simulink model "INCMPPT"  (R2014b)
settings: Solver=ode45  StartTime=0.0  StopTime=2  RelTol=1e-3
undefined symbols (not defined in the file or in its folder): sigbuilder_block
libraries: powerlib x14, powerlib_meascontrol x1
settings Model: Creator=nitukeee  LastModifiedBy=nitukeee

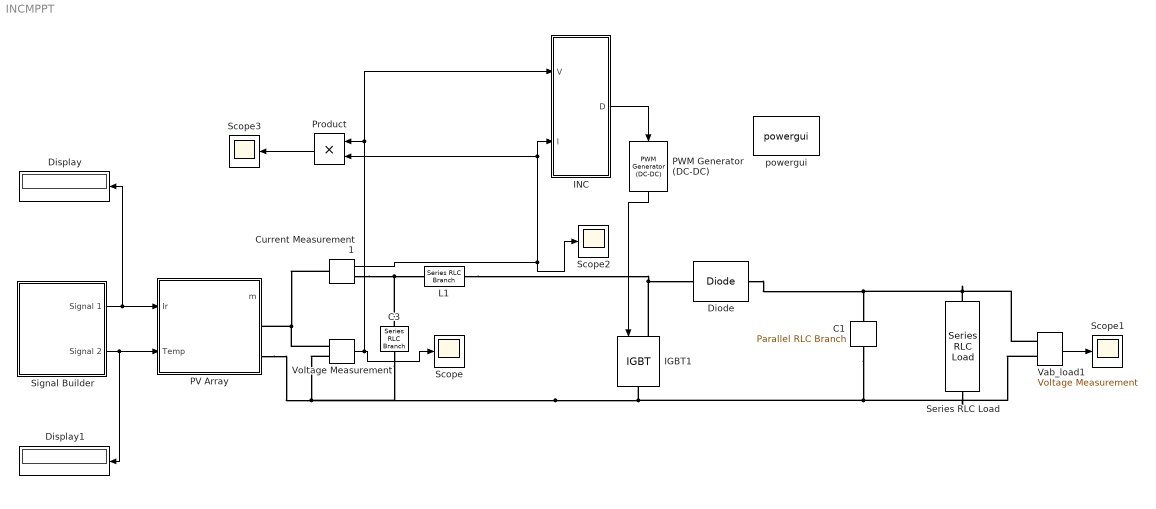
== system INCMPPT ==
  C1 : powerlib/Elements/Parallel RLC Branch  LConnTagsString=a  RConnTagsString=__new0  BranchType=C  Resistance=1  Inductance=1e-3  SetiL0=off  InitialCurrent=0  Capacitance=12000e-6  Setx0=off  InitialVoltage=0  Measurements=None
  C3 : powerlib/Elements/Series RLC Branch  LConnTagsString=__new0  RConnTagsString=__new0  BranchType=C  Resistance=1  Inductance=1e-3  SetiL0=off  InitialCurrent=0  Capacitance=100e-6  Setx0=off  InitialVoltage=0  Measurements=None
  Current Measurement1 : powerlib/Measurements/Current Measurement  PhasorSimulation=off  OutputType=Complex  PSBequivalent=0
  Diode : powerlib/Power Electronics/Diode  Ron=0.001  Lon=0  Vf=0.8  IC=0  UseSnubber=off  Rs=500  Cs=250e-9  Measurements=off
  Display : Display
  Display1 : Display
  IGBT1 : powerlib/Power Electronics/IGBT  Ron=0.001  Lon=0  Vf=1  Tf=1e-6  Tt=2e-6  IC=0  Rs=1e5  Cs=inf  Measurements=off
  INC : Subsystem
  L1 : powerlib/Elements/Series RLC Branch  LConnTagsString=__new0  RConnTagsString=__new0  BranchType=RL  Resistance=0.005  Inductance=0.005  SetiL0=off  InitialCurrent=0  Capacitance=1e-6  Setx0=off  InitialVoltage=0  Measurements=None
  PV Array : Subsystem  mask(PV array){ModuleType=SunPower SPR-305-WHT, Ncell=96, Nser=5, Npar=66, Voc=64.2, Isc=5.96, Vm=54.7, Im=5.58, TempC_Voc=-0.177, TempC_Isc=0.003516, TempC_Vmp=-0.186, TempC_Imp=-0.00212, Qd=1.25, Temperature=[0   25   50   75  100], Iph_Temp=[5.9045      5.9606      6.0494      6.1386      6.2292], Isat_Temp=[1.6236e-10  5.2622e-09  9.8888e-08  1.2201e-06  1.0769e-05], Rp_Temp=[1723.2701      819.13001       313.3225      186.86379      130.70398], Rs_Temp=[0.10187    0.083029    0.075997    0.085738      0.1163], PlotVI_module=off, PlotVI_array=off, PlotVI_array_Temp=off, Ts=1e-6}
      mask prompts: ModuleType "Module type:"; Ncell "Number of cells per module:"; Nser "Number of series-connected  modules per string (Nser):"; Npar "Number of parallel strings (Npar):"; Voc "Open circuit voltage  Voc (V):"; Isc "Short-circuit current Isc (A):"; Vm "Voltage at maximum power point Vmp (V):"; Im "Current at maximum power point Imp (A):"; TempC_Voc "Temperature coefficient of Voc (V/deg.C)"; TempC_Isc "Temperature coefficient of Isc (A/deg.C)"; TempC_Vmp "Temperature coefficient of Vmp (V/deg.C)"; TempC_Imp "Temperature coefficient of Imp (A/deg.C"; Qd "Diode Quality factor"; Temperature "Cell temperature (degrees C)"; Iph_Temp "Photo-current source Iph  (A):"; Isat_Temp "Diode saturation current Isat (A):"; Rp_Temp "Parallel resistance Rp (ohms):"; Rs_Temp "Series resistance Rs (ohms):"; PlotVI_module "Display  I-V and  P-V characteristics of one module at 25 deg.C"; PlotVI_array "Display  I-V and  P-V characteristics of array at 25 deg.C"; PlotVI_array_Temp "Display  I-V and  P-V char. of array at 100W/m^2  for specified temperatures"; Ts "Sample time"
      mask help:
      | Model a PV array.
      |
      | PV array consists of Npar strings of modules connected in parallel, each string consisting of Nser modules connected in series.
      |
      | Input 1 = Sun irradiance (W/m^2)
      | Input 2 = Cell temperature (deg.C))
      |
      | Module specifications provided by manufacturer (Voc, Isc, Vmp, Imp) as well as temperature coefficients are listed under 'Module' Tab.
      | The four PV model parameters for one module (photo-generated current Iph, diode saturation current Isat, parallel resistance Rp and  series resistance Rs) are listed under the 'Model' Tab. These parameters are adusted to fit Voc, Isc, Vmp, Imp at specied cell temperatures listed under 'Module' Tab and assuming a given "diode quality factor" (Qd) for the semiconductor.
      |
      | Select a 'Module type' and then press Apply to see module parameters.
      | Note: Module characteristics are extracted from NREL System Advisor Model.
      mask init:
      | BlockName=gcb;
      | 
      | % Solar Modules Specifications
      | %=============================
      | %
      | Type=1;
      | SolarModuleSpec(Type).Desc= 'Kyocera KD135GX-LP';
      | SolarModuleSpec(Type).nCells= 36;
      | SolarModuleSpec(Type).Voc= 22.0999;
      | SolarModuleSpec(Type).Isc= 8.36955;
      | SolarModuleSpec(Type).Vmp= 17.7;
      | SolarModuleSpec(Type).Imp= 7.62959;
      | SolarModuleSpec(Type).TempC_Voc= -0.08;
      | SolarModuleSpec(Type).TempC_Isc= 0.005022;
      | SolarModuleSpec(Type).TempC_Vmp= -0.082;
      | SolarModuleSpec(Type).TempC_Imp= -0.001068;
      | SolarModuleSpec(Type).TempC= [0   25   50   75  100];
      | SolarModuleSpec(Type).Qd= 1.25;
      | SolarModuleSpec(Type).Iph= [8.2548      8.3863      8.5179      8.6475      8.7657];
      | SolarModuleSpec(Type).Isat= [1.0452e-09  4.0088e-08  8.7854e-07   1.246e-05  0.00012585];
      | SolarModuleSpec(Type).Rp= [124.2147      80.21788      61.82143      57.59975       93.2949];
      | SolarModuleSpec(Type).Rs= [0.16273     0.16086     0.16567     0.17914     0.20462];
      | SolarModuleSpec(Type).VT= [1.0586      1.1555      1.2525      1.3494      1.4463];
      | 
      | Type=2;
      | SolarModuleSpec(Type).Desc= 'Kyocera KD205GX-LP';
      | SolarModuleSpec(Type).nCells= 54;
      | SolarModuleSpec(Type).Voc= 33.1999;
      | SolarModuleSpec(Type).Isc= 8.35955;
      | SolarModuleSpec(Type).Vmp= 26.6;
      | SolarModuleSpec(Type).Imp= 7.70959;
      | SolarModuleSpec(Type).TempC_Voc= -0.12;
      | SolarModuleSpec(Type).TempC_Isc= 0.005016;
      | SolarModuleSpec(Type).TempC_Vmp= -0.123;
      | SolarModuleSpec(Type).TempC_Imp= -0.001079;
      | SolarModuleSpec(Type).TempC= [0   25   50   75  100];
      | SolarModuleSpec(Type).Qd= 1.5;
      | SolarModuleSpec(Type).Iph= [8.2611      8.3642      8.4897      8.6397      8.8494];
      | SolarModuleSpec(Type).Isat= [4.6184e-08  9.7399e-07  1.2856e-05  0.00011784  0.00080899];
      | SolarModuleSpec(Type).Rp= [1053.4598       1010.571      746.03259      733.82072      575.51725];
      | SolarModuleSpec(Type).Rs= [0.16179     0.15945     0.16818     0.19126     0.23373];
      | SolarModuleSpec(Type).VT= [1.9055      2.0799      2.2544      2.4289      2.6034];
      | 
      | Type=3;
      | SolarModuleSpec(Type).Desc= 'Mitsubishi PV-UD190MF5';
      | SolarModuleSpec(Type).nCells= 50;
      | SolarModuleSpec(Type).Voc= 30.8006;
      | SolarModuleSpec(Type).Isc= 8.23289;
      | SolarModuleSpec(Type).Vmp= 24.6999;
      | SolarModuleSpec(Type).Imp= 7.71272;
      | SolarModuleSpec(Type).TempC_Voc= -0.105;
      | SolarModuleSpec(Type).TempC_Isc= 0.004446;
      | SolarModuleSpec(Type).TempC_Vmp= -0.109;
      | SolarModuleSpec(Type).TempC_Imp= -0.0007713;
      | SolarModuleSpec(Type).TempC= [0   25   50   75  100];
      | SolarModuleSpec(Type).Qd= 1.25;
      | SolarModuleSpec(Type).Iph= [8.1758      8.2585      8.3644      8.4965      8.6704];
      | SolarModuleSpec(Type).Isat= [1.0882e-09  3.8061e-08  7.7001e-07  1.0166e-05  9.5622e-05];
      | SolarModuleSpec(Type).Rp= [760.17338      1011.1501      920.18116      953.25748       1044.703];
      | SolarModuleSpec(Type).Rs= [0.22154      0.2231     0.23302     0.25351     0.28829];
      | SolarModuleSpec(Type).VT= [1.4703      1.6049      1.7395      1.8742      2.0088];
      | 
      | Type=4;
      | SolarModuleSpec(Type).Desc= 'Sanyo HIP-225HDE1';
      | SolarModuleSpec(Type).nCells= 60;
      | SolarModuleSpec(Type).Voc= 41.7984;
      | SolarModuleSpec(Type).Isc= 7.13383;
      | SolarModuleSpec(Type).Vmp= 33.9;
      | SolarModuleSpec(Type).Imp= 6.63419;
      | SolarModuleSpec(Type).TempC_Voc= -0.105;
      | SolarModuleSpec(Type).TempC_Isc= 0.00214;
      | SolarModuleSpec(Type).TempC_Vmp= -0.101;
      | SolarModuleSpec(Type).TempC_Imp= -0.0006634;
      | SolarModuleSpec(Type).TempC= [0   25   50   75  100];
      | SolarModuleSpec(Type).Qd= 1.75;
      | SolarModuleSpec(Type).Iph= [7.1125      7.1668      7.2277      7.3002      7.3835];
      | SolarModuleSpec(Type).Isat= [1.0956e-07   1.322e-06  1.0873e-05  6.6227e-05  0.00031754];
      | SolarModuleSpec(Type).Rp= [1677.488      1798.4952      1967.0424      1956.9124      2053.1618];
      | SolarModuleSpec(Type).Rs= [0.19173     0.14196     0.10096    0.069476    0.049098];
      | SolarModuleSpec(Type).VT= [2.47      2.6962      2.9224      3.1486      3.3748];
      | 
      | Type=5;
      | SolarModuleSpec(Type).Desc= 'SunPower SPR-305-WHT';
      | SolarModuleSpec(Type).nCells= 96;
      | SolarModuleSpec(Type).Voc= 64.2;
      | SolarModuleSpec(Type).Isc= 5.96;
      | SolarModuleSpec(Type).Vmp= 54.7;
      | SolarModuleSpec(Type).Imp= 5.58;
      | SolarModuleSpec(Type).TempC_Voc= -0.177;
      | SolarModuleSpec(Type).TempC_Isc= 0.003516;
      | SolarModuleSpec(Type).TempC_Vmp= -0.186;
      | SolarModuleSpec(Type).TempC_Imp= -0.00212;
      | SolarModuleSpec(Type).TempC= [0   25   50   75  100];
      | SolarModuleSpec(Type).Qd= 1.25;
      | SolarModuleSpec(Type).Iph= [5.9045      5.9606      6.0494      6.1386      6.2292];
      | SolarModuleSpec(Type).Isat= [1.6236e-10  5.2622e-09  9.8888e-08  1.2201e-06  1.0769e-05];
      | SolarModuleSpec(Type).Rp= [1723.2701      819.13001       313.3225      186.86379      130.70398];
      | SolarModuleSpec(Type).Rs= [0.10187    0.083029    0.075997    0.085738      0.1163];
      | SolarModuleSpec(Type).VT= [2.8229      3.0814      3.3399      3.5984      3.8569];
      | 
      | Type=6;
      | SolarModuleSpec(Type).Desc= 'Suntech STP270S-24_Vb';
      | SolarModuleSpec(Type).nCells= 72;
      | SolarModuleSpec(Type).Voc= 44.4999;
      | SolarModuleSpec(Type).Isc= 8.19978;
      | SolarModuleSpec(Type).Vmp= 35;
      | SolarModuleSpec(Type).Imp= 7.70979;
      | SolarModuleSpec(Type).TempC_Voc= -0.1504;
      | SolarModuleSpec(Type).TempC_Isc= 0.004969;
      | SolarModuleSpec(Type).TempC_Vmp= -0.1567;
      | SolarModuleSpec(Type).TempC_Imp= 0.0001234;
      | SolarModuleSpec(Type).TempC= [0   25   50   75  100];
      | SolarModuleSpec(Type).Qd= 1.25;
      | SolarModuleSpec(Type).Iph= [8.1345      8.2466      8.3792      8.5437      8.7583];
      | SolarModuleSpec(Type).Isat= [1.0212e-09   3.569e-08  7.2273e-07  9.5489e-06  8.9954e-05];
      | SolarModuleSpec(Type).Rp= [1505.3115      1827.4593      2300.9307      2164.0121      1763.1975];
      | SolarModuleSpec(Type).Rs= [0.4218     0.42722     0.44553     0.48023      0.5376];
      | SolarModuleSpec(Type).VT= [2.1172      2.3111      2.5049      2.6988      2.8927];
      | 
      | Type=7;
      | SolarModuleSpec(Type).Desc= 'Canadian Solar CS5P-220M';
      | SolarModuleSpec(Type).nCells= 96;
      | SolarModuleSpec(Type).Voc= 59.2618;
      | SolarModuleSpec(Type).Isc= 5.09261;
      | SolarModuleSpec(Type).Vmp= 48.3159;
      | SolarModuleSpec(Type).Imp= 4.54758;
      | SolarModuleSpec(Type).TempC_Voc= -0.217;
      | SolarModuleSpec(Type).TempC_Isc= 0.002022;
      | SolarModuleSpec(Type).TempC_Vmp= -0.2355;
      | SolarModuleSpec(Type).TempC_Imp= 0.0008231;
      | SolarModuleSpec(Type).TempC= [0   25   50   75  100];
      | SolarModuleSpec(Type).Qd= 1.5;
      | SolarModuleSpec(Type).Iph= [5.046       5.098      5.1493      5.1959      5.3427];
      | SolarModuleSpec(Type).Isat= [2.4207e-08  5.3103e-07  7.2907e-06  6.9747e-05  0.00049283];
      | SolarModuleSpec(Type).Rp= [222.52442      235.76261      303.25525      1307.0023      2378.4408];
      | SolarModuleSpec(Type).Rs= [0.17441     0.24807     0.36157     0.52616      0.7509];
      | SolarModuleSpec(Type).VT= [3.3875      3.6977      4.0079      4.3181      4.6283];
      | 
      | Type=8;
      | SolarModuleSpec(Type).Desc= 'BP Solar SX3190';
      | SolarModuleSpec(Type).nCells= 50;
      | SolarModuleSpec(Type).Voc= 30.6021;
      | SolarModuleSpec(Type).Isc= 8.51029;
      | SolarModuleSpec(Type).Vmp= 24.3003;
      | SolarModuleSpec(Type).Imp= 7.82945;
      | SolarModuleSpec(Type).TempC_Voc= -0.111;
      | SolarModuleSpec(Type).TempC_Isc= 0.005532;
      | SolarModuleSpec(Type).TempC_Vmp= -0.114;
      | SolarModuleSpec(Type).TempC_Imp= -0.001566;
      | SolarModuleSpec(Type).TempC= [0   25   50   75  100];
      | SolarModuleSpec(Type).Qd= 1.25;
      | SolarModuleSpec(Type).Iph= [8.3797      8.5214       8.667      8.8096      8.9362];
      | SolarModuleSpec(Type).Isat= [1.1494e-09  4.3763e-08   9.524e-07  1.3432e-05  0.00013518];
      | SolarModuleSpec(Type).Rp= [479.1668      189.6748      120.6956      107.8176      267.7255];
      | SolarModuleSpec(Type).Rs= [0.24905     0.24841     0.25704     0.27792     0.31611];
      | SolarModuleSpec(Type).VT= [1.4703      1.6049      1.7395      1.8742      2.0088];
      | 
      | Type=9;
      | SolarModuleSpec(Type).Desc= 'First Solar FS-272';
      | SolarModuleSpec(Type).nCells= 116;
      | SolarModuleSpec(Type).Voc= 94.5738;
      | SolarModuleSpec(Type).Isc= 1.18103;
      | SolarModuleSpec(Type).Vmp= 70.558;
      | SolarModuleSpec(Type).Imp= 1.01088;
      | SolarModuleSpec(Type).TempC_Voc= -0.269;
      | SolarModuleSpec(Type).TempC_Isc= 0.0005433;
      | SolarModuleSpec(Type).TempC_Vmp= -0.206;
      | SolarModuleSpec(Type).TempC_Imp= -0.0003538;
      | SolarModuleSpec(Type).TempC= [0   25   50   75  100];
      | SolarModuleSpec(Type).Qd= 3;
      | SolarModuleSpec(Type).Iph= [1.1706      1.1841      1.1969       1.209      1.2204];
      | SolarModuleSpec(Type).Isat= [4.7807e-06   2.871e-05  0.00013082  0.00048055    0.001489];
      | SolarModuleSpec(Type).Rp= [2555.993      1859.5401      1459.3976      1213.5712      1072.4965];
      | SolarModuleSpec(Type).Rs= [6.9861      4.7977      2.7078     0.74048           0];
      | SolarModuleSpec(Type).VT= [8.1864      8.93607      9.68574      10.4354      11.1851];
      | 
      | Type=10;
      | SolarModuleSpec(Type).Desc= 'SunPower 128-cell Module';
      | SolarModuleSpec(Type).nCells= 128;
      | SolarModuleSpec(Type).Voc= 85.2983;
      | SolarModuleSpec(Type).Isc= 5.8675;
      | SolarModuleSpec(Type).Vmp= 72.8992;
      | SolarModuleSpec(Type).Imp= 5.48769;
      | SolarModuleSpec(Type).TempC_Voc= -0.2664;
      | SolarModuleSpec(Type).TempC_Isc= 0.001837;
      | SolarModuleSpec(Type).TempC_Vmp= -0.276;
      | SolarModuleSpec(Type).TempC_Imp= -0.00169;
      | SolarModuleSpec(Type).TempC= [0   25   50   75  100];
      | SolarModuleSpec(Type).Qd= 1.5;
      | SolarModuleSpec(Type).Iph= [5.8403      5.8693      5.9126      5.9583      6.0069];
      | SolarModuleSpec(Type).Isat= [8.3639e-09  1.7905e-07  2.3847e-06  2.1965e-05  0.00015113];
      | SolarModuleSpec(Type).Rp= [3739.8323      3390.2471      1695.8516      1327.4043      1910.4252];
      | SolarModuleSpec(Type).Rs= [0  0  0  0  0];
      | SolarModuleSpec(Type).VT= [4.5166      4.9302      5.3439      5.7575      6.1711];
      | 
      | 
      | %-------------------------------------------------------------------------
      | 
      | Type=strmatch(ModuleType,char(SolarModuleSpec.Desc));
      | 
      | % Write module prameters inside mask
      | %===================================
      | set_param(BlockName,'Ncell',num2str(SolarModuleSpec(Type).nCells));
      | set_param(BlockName,'Voc',num2str(SolarModuleSpec(Type).Voc));
      | set_param(BlockName,'Isc',num2str(SolarModuleSpec(Type).Isc));
      | set_param(BlockName,'Vm',num2str(SolarModuleSpec(Type).Vmp));
      | set_param(BlockName,'Im',num2str(SolarModuleSpec(Type).Imp));
      | set_param(BlockName,'TempC_Voc',num2str(SolarModuleSpec(Type).TempC_Voc));
      | set_param(BlockName,'TempC_Isc',num2str(SolarModuleSpec(Type).TempC_Isc));
      | set_param(BlockName,'TempC_Vmp',num2str(SolarModuleSpec(Type).TempC_Vmp));
      | set_param(BlockName,'TempC_Imp',num2str(SolarModuleSpec(Type).TempC_Imp));
      | 
      | set_param(BlockName,'Qd',num2str(SolarModuleSpec(Type).Qd));
      | 
      | set_param(BlockName,'Temperature',['[',num2str(SolarModuleSpec(Type).TempC),']']);
      | set_param(BlockName,'Iph_Temp',['[',num2str(SolarModuleSpec(Type).Iph),']']);
      | set_param(BlockName,'Isat_Temp',['[',num2str(SolarModuleSpec(Type).Isat),']']);
      | set_param(BlockName,'Rp_Temp',['[',num2str(SolarModuleSpec(Type).Rp),']']);
      | set_param(BlockName,'Rs_Temp',['[',num2str(SolarModuleSpec(Type).Rs),']']);
      | 
      | TC=25; % standard test temperature (deg. C)
      | T=273+TC; %(Kelvin)
      | nT=find(SolarModuleSpec(Type).TempC==TC);
      | 
      | % Array model parameters
      | %=======================
      | % Qd=SolarModuleSpec(Type).Qd;
      | % k= 1.3806e-23; % Boltzman constant (J.K^-1)
      | % q=1.6022e-19;  % electron charge  (C)
      | % VT=k*T/q*nCells*Qd;
      | VT=SolarModuleSpec(Type).VT(nT);Iph=SolarModuleSpec(Type).Iph(nT); 
      | 
      | TempC=SolarModuleSpec(Type).TempC;
      | Iph_array=SolarModuleSpec(Type).Iph*Npar;
      | Isat_array=SolarModuleSpec(Type).Isat*Npar;
      | VT_array=SolarModuleSpec(Type).VT*Nser;
      | Rs_array=SolarModuleSpec(Type).Rs*Nser/Npar;
      | Rp_array=SolarModuleSpec(Type).Rp*Nser/Npar;
      | 
      | % Used to determine initial value of Boost Control (MPPT)
      | % assignin('base','Vm_Init',Vm*Nser);
      | %
      | % Plot module and array I-V & P-V characteristics for different irradiances
      | % =========================================================================
      | if PlotVI_module || PlotVI_array 
      |     Voc=SolarModuleSpec(Type).Voc; 
      |     Isc=SolarModuleSpec(Type).Isc; 
      |     Vm=SolarModuleSpec(Type).Vmp;  
      |     Im=SolarModuleSpec(Type).Imp;
      |     
      |     load_system('PV_model_Param');
      |     
      |     assignin('base','Voc',Voc);
      |     assignin('base','Isc',Isc);
      |     assignin('base','Rs',SolarModuleSpec(Type).Rs(nT));
      |     assignin('base','Rp',SolarModuleSpec(Type).Rp(nT));
      |     assignin('base','Isat',SolarModuleSpec(Type).Isat(nT));
      |     assignin('base','VT',SolarModuleSpec(Type).VT(nT));
      |    
      |     if PlotVI_module,
      |         F1=figure('Name','I-V and P-V characteristics of one module at 25 deg.C');  
      |     end
      |     if PlotVI_array
      |         F2=figure('Name','I-V and P-V characteristics of array at 25 deg.C'); 
      |     end
      | 
      |     for ksun=1:-0.25:0.25
      |         assignin('base','Iph',SolarModuleSpec(Type).Iph(nT)*ksun);
      |         sim('PV_model_Param');
      |         n=find(I_PV>=0);
      |         I_PV=I_PV(n);
      |         V_PV=V_PV(n);
      |         P_PV=V_PV.*I_PV;
      |         
      |         % Plot I-V & P-V characteristics of one module
      |         %=============================================
      |         if PlotVI_module
      |             figure(F1);
      |             subplot(211)
      |             if ksun==1
      |                 plot(V_PV,I_PV,'b',[0  Vm Voc], [Isc Im 0],'ro')
      |                 text(Voc/15,Isc*1.1,'1 kW/m^2')
      |                 hold on
      |                 grid
      |             else
      |                 plot(V_PV,I_PV,'--m')
      |                 text(Voc/15, Isc*(ksun+0.1) , sprintf('%g kW/m^2',ksun))
      |             end
      | 
      |             subplot(212) 
      |             if ksun==1
      |                 plot(V_PV,P_PV,'b',[0  Vm Voc], [0 Im*Vm 0],'ro')
      |                 text(Vm*1.02,Vm*Im,'1 kW/m^2')
      |                 hold on
      |                 grid
      |             else
      |                 n= find(P_PV==max(P_PV));
      |                 plot(V_PV,P_PV,'--m', V_PV(n) , P_PV(n),'mo')
      |                 text(Vm*1.02, Vm*Im*ksun, sprintf('%g kW/m^2',ksun))
      |             end
      |             subplot(211)
      |             ylabel('Current (A)')
      |             xlabel('Voltage (V)')
      |             title(sprintf('Module type: %s',SolarModuleSpec(Type).Desc))
      |             axis_xy=axis;
      |             axis_xy(4)=Isc*1.2;
      |             axis(axis_xy);
      |             
      |             subplot(212)
      |             ylabel('Power (W)')
      |             xlabel('Voltage (V)')
      |             axis_xy=axis;
      |             axis_xy(4)=Vm*Im*1.2;
      |             axis(axis_xy);
      |                   
      |             set_param(BlockName,'PlotVI_module', 'off')
      |         end
      |         
      |         % Plot I-V & P-V characteristics of array
      |         %========================================
      |         if PlotVI_array
      |             figure(F2);
      |             subplot(211)
      |             if ksun==1
      |                 plot(V_PV*Nser,I_PV*Npar,'b',[0  Vm Voc]*Nser, [Isc Im 0]*Npar,'ro')
      |                 text(Voc/15*Nser,Isc*1.1*Npar,'1 kW/m^2')
      |                 hold on
      |                 grid
      |             else
      |                 plot(V_PV*Nser,I_PV*Npar,'--m')
      |                 text(Voc*Nser/15, Isc*Npar*(ksun+0.1) , sprintf('%g kW/m^2',ksun))
      |             end
      |            
      |             subplot(212)
      |             if ksun==1
      |                 plot(V_PV*Nser,P_PV*Nser*Npar,'b',[0  Vm Voc]*Nser, [0 Im*Vm 0]*Nser*Npar,'ro')
      |                 text(Vm*Nser*1.02,Vm*Im*Nser*Npar,'1 kW/m^2')
      |                 hold on
      |                 grid
      |             else
      |                 n= find(P_PV==max(P_PV));
      |                 plot(V_PV*Nser,P_PV*Nser*Npar,'--m', V_PV(n)*Nser , P_PV(n)*Nser*Npar,'mo')
      |                 text(Vm*Nser*1.02, Vm*Im*Nser*Npar*ksun, sprintf('%g kW/m^2',ksun))
      |             end 
      |             subplot(211)
      |             ylabel('Current (A)')
      |             xlabel('Voltage (V)')
      |             title(sprintf('Array type: %s; %d series modules; %d parallel strings',SolarModuleSpec(Type).Desc,Nser,Npar));
      |             axis_xy=axis;
      |             axis_xy(4)=Isc*Npar*1.2;
      |             axis(axis_xy);
      |             
      |             subplot(212)
      |             ylabel('Power (W)')
      |             xlabel('Voltage (V)')
      |             xis_xy=axis;
      |             axis_xy(4)=Vm*Im*Nser*Npar*1.2;
      |             axis(axis_xy);
      |             
      |             set_param(BlockName,'PlotVI_array', 'off')
      |         end
      |         
      |     end  
      | end
      | 
      | %%  Plot array V-I & P_V characteristics for different temperatures
      | % =================================================================
      | if PlotVI_array_Temp
      |     F3=figure('Name',' I-V and P-V characteristics of array at 1000 W/m^2');
      |     load_system('PV_model_Param');
      |     for ktemp=1:length(TempC)
      |         DeltaT=TempC(ktemp)-25;
      |         Voc=SolarModuleSpec(Type).Voc + SolarModuleSpec(Type).TempC_Voc*DeltaT;
      |         Isc=SolarModuleSpec(Type).Isc + SolarModuleSpec(Type).TempC_Isc*DeltaT;
      |         Vm=SolarModuleSpec(Type).Vmp  + SolarModuleSpec(Type).TempC_Vmp*DeltaT;
      |         Im=SolarModuleSpec(Type).Imp  + SolarModuleSpec(Type).TempC_Imp*DeltaT;
      | 
      |         assignin('base','Voc',Voc)
      |         assignin('base','Isc',Isc)
      |         assignin('base','Iph',SolarModuleSpec(Type).Iph(ktemp));
      |         assignin('base','Isat',SolarModuleSpec(Type).Isat(ktemp));
      |         assignin('base','Rs',SolarModuleSpec(Type).Rs(ktemp));
      |         assignin('base','Rp',SolarModuleSpec(Type).Rp(ktemp));
      |         assignin('base','VT',SolarModuleSpec(Type).VT(ktemp));
      |         
      |         sim('PV_model_Param');
      |         n=find(I_PV>=0);
      |         I_PV=I_PV(n);
      |         V_PV=V_PV(n);
      |         P_PV=V_PV.*I_PV;
      | 
      |         subplot(211)
      |         if TempC(ktemp)==25
      |             plot(V_PV*Nser,I_PV*Npar,'b',[0  Vm Voc]*Nser, [Isc Im 0]*Npar,'ro')
      |             text(Voc*Nser*0.95, Isc*Npar/10*(1+ktemp) , sprintf('%g ^oC',TempC(ktemp)))
      |             %hold on
      |             grid
      |         else
      |             plot(V_PV*Nser,I_PV*Npar,'--m',[0  Vm Voc]*Nser, [Isc Im 0]*Npar,'mo')
      |             text(Voc*Nser*0.95, Isc*Npar/10*(1+ktemp) , sprintf('%g ^oC',TempC(ktemp)))
      |         end
      |         if ktemp==1, hold on; end
      | 
      |         subplot(212) 
      |         if TempC(ktemp)==25
      |             plot(V_PV*Nser,P_PV*Nser*Npar,'b',[0  Vm Voc]*Nser, [0 Im*Vm 0]*Nser*Npar,'ro')
      |             text(Vm*Nser, 0.9*Vm*Im*Nser*Npar , sprintf('%g ^oC',TempC(ktemp)))
      |             %hold on
      |             grid
      |         else
      |             n= find(P_PV==max(P_PV));
      |             plot(V_PV*Nser,P_PV*Nser*Npar,'--m', V_PV(n)*Nser , P_PV(n)*Nser*Npar,'mo')
      |             text(Vm*Nser, 0.9*Vm*Im*Nser*Npar , sprintf('%g ^oC',TempC(ktemp)))
      |         end
      |         if ktemp==1, hold on; end
      |     end
      |         
      |     subplot(211)
      |     ylabel('Current (A)')
      |     xlabel('Voltage (V)')
      |     title(sprintf('Array type: %s; %d series modules; %d parallel strings',SolarModuleSpec(Type).Desc,Nser,Npar));
      |     subplot(212)
      |     ylabel('Power (W)')
      |     xlabel('Voltage (V)')
      |     set_param(BlockName,'PlotVI_array_Temp', 'off')
      | end
      mask TypeOptions ModuleType: BP Solar SX3190 | Canadian Solar CS5P-220M | First Solar FS-272 | Kyocera KD135GX-LP | Kyocera KD205GX-LP | Mitsubishi PV-UD190MF5 | Sanyo HIP-225HDE1 | SunPower SPR-305-WHT | SunPower SPR-400-WHT | Suntech STP270S-24_Vb
      mask Display: image(imread('panel.jpg'))
  PWM Generator (DC-DC) : powerlib_meascontrol/Pulse & Signal Generators/PWM Generator (DC-DC)  Fsw=5000  Ts=0
  Product : Product
  Scope{,1..3} (4 alike) : Scope
      Scope settings: YMin=50  YMax=350
      Scope1 settings: YMin=0  YMax=500
      Scope2 settings: YMin=-0.0381367  YMax=400  SaveName=ScopeData2
      Scope3 settings: YMin=-60000  YMax=120000  SaveName=ScopeData3
  Series RLC Load : powerlib/Elements/Series RLC Load  LConnTagsString=a  RConnTagsString=__new0  NominalVoltage=500  NominalFrequency=50  ActivePower=100e3  InductivePower=0  CapacitivePower=0  Setx0=off  InitialVoltage=0  SetiL0=off  InitialCurrent=0  Measurements=None
  Signal Builder : Subsystem  Tag=STV Subsys  LoadFcn=sigbuilder_block('load');  StartFcn=sigbuilder_block('start');  StopFcn=sigbuilder_block('stop');  ClipboardFcn=sigbuilder_block('clipboard');  mask(Sigbuilder block){}
      mask help: Simulink:masks:SigbuilderBlock_MD
      mask init:
      | if ~strcmp(get_param(bdroot(gcbh),'SimulationStatus'),'stopped') tuvar = sigbuilder_block('maskInit'); end
      settings: CopyFcn=sigbuilder_block('copy');  DeleteFcn=sigbuilder_block('delete');  ModelCloseFcn=sigbuilder_block('modelClose');  PreSaveFcn=sigbuilder_block('preSave');  PauseFcn=sigbuilder_block('pause');  ContinueFcn=sigbuilder_block('continue');  NameChangeFcn=sigbuilder_block('namechange');  OpenFcn=sigbuilder_block('open',[437.6 199.2 550.4 400 ]);  CloseFcn=sigbuilder_block('close');
      mask Display: plot(0, 0, 100, 100,[2, 2, 32, 32, 2], [68, 8, 8, 68, 68],[32, 2], [38, 38], [32, 19, 2],[53, 60, 44], [32, 17, 17, 2],[16, 16, 31, 31]);txt = getActiveGroup(gcbh);text(2, 100, txt,'verticalAlignment', 'top');
  Vab_load1 : powerlib/Measurements/Voltage Measurement  Tag=PoWeRsYsTeMmEaSuReMeNt  PhasorSimulation=off  OutputType=Complex  PSBequivalent=0
  Voltage Measurement : powerlib/Measurements/Voltage Measurement  PhasorSimulation=off  OutputType=Complex  PSBequivalent=0
  powergui : powerlib/powergui  Priority=1  SimulationMode=Discrete  SolverType=Tustin/Backward Euler (TBE)  SampleTime=1e-06  frequency=60  SPID=off  DisableSnubberDevices=off  DisableRonSwitches=off  DisableVfSwitches=off  SwTol=0  DisplayEquations=off  Interpol=off  methode=off  Ts=100  frequencyindice=0  Pbase=100e6  ErrMax=1e-4  Iterations=50  UnitsV=kV  UnitsW=MW  FunctionMessages=off  echomessages=off  HookPort=off  EnableUseOfTLC=off  x0status=blocks  RestoreLinks=warning  ResistiveCurrentMeasurement=off  Frange=[0:2:500]  Ylog=off  Xlog=on  ShowGrid=off  save=off  variable=ZData  structure=0  ZoomFFT=off  StartTime=0.0  cycles=1  DisplayStyle=1  fundamental=60  FreqAxis=off  MaxFrequency=1000  frequencyindicesteady=1  RmsSteady=1  display=off
  wires:
  Current Measurement1/1 -> Scope2/1, Product/2, INC/2(I)
  Voltage Measurement/1 -> Product/1, INC/1(V), Scope/1
  Vab_load1/1 -> Scope1/1
  Product/1 -> Scope3/1
  Signal Builder/1(Signal 1) -> Display/1, PV Array/1(Ir)
  Signal Builder/2(Signal 2) -> Display1/1, PV Array/2(Temp)
  PWM Generator (DC-DC)/1 -> IGBT1/1
  INC/1(D) -> PWM Generator (DC-DC)/1
  connections:
  PV Array/RConn2 -- C3/RConn1 -- IGBT1/RConn1 -- C1/RConn1 -- Vab_load1/LConn2 -- Series RLC Load/RConn1 -- Voltage Measurement/LConn2
  Vab_load1/LConn1 -- Series RLC Load/LConn1 -- Diode/RConn1 -- C1/LConn1
  C3/LConn1 -- Current Measurement1/RConn1 -- L1/LConn1
  IGBT1/LConn1 -- L1/RConn1 -- Diode/LConn1
  Voltage Measurement/LConn1 -- Current Measurement1/LConn1 -- PV Array/RConn1

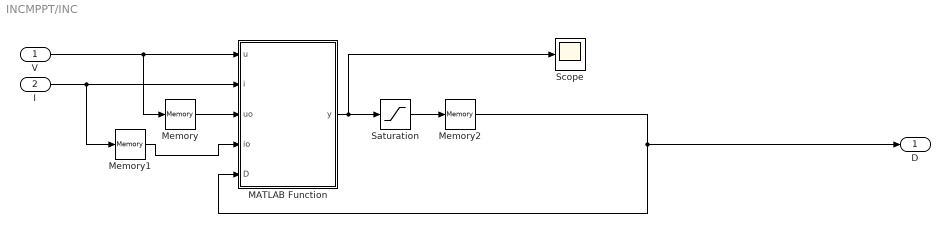
== system INCMPPT/INC ==
  V : Inport
  I : Inport  Port=2
  MATLAB Function : MATLAB Function  TreatAsAtomicUnit=on
  Memory : Memory  InheritSampleTime=on
  Memory1 : Memory  InheritSampleTime=on
  Memory2 : Memory  InheritSampleTime=on
  Saturation : Saturate  UpperLimit=0.9  LowerLimit=0
  Scope : Scope
      settings: YMin=-0.5  YMax=2  SaveName=ScopeData4
  D : Outport
  wires:
  Memory/1 -> MATLAB Function/3(uo)
  Saturation/1 -> Memory2/1
  V/1 -> Memory/1, MATLAB Function/1(u)
  Memory1/1 -> MATLAB Function/4(io)
  I/1 -> Memory1/1, MATLAB Function/2(i)
  Memory2/1 -> D/1, MATLAB Function/5(D)
  MATLAB Function/1(y) -> Scope/1, Saturation/1

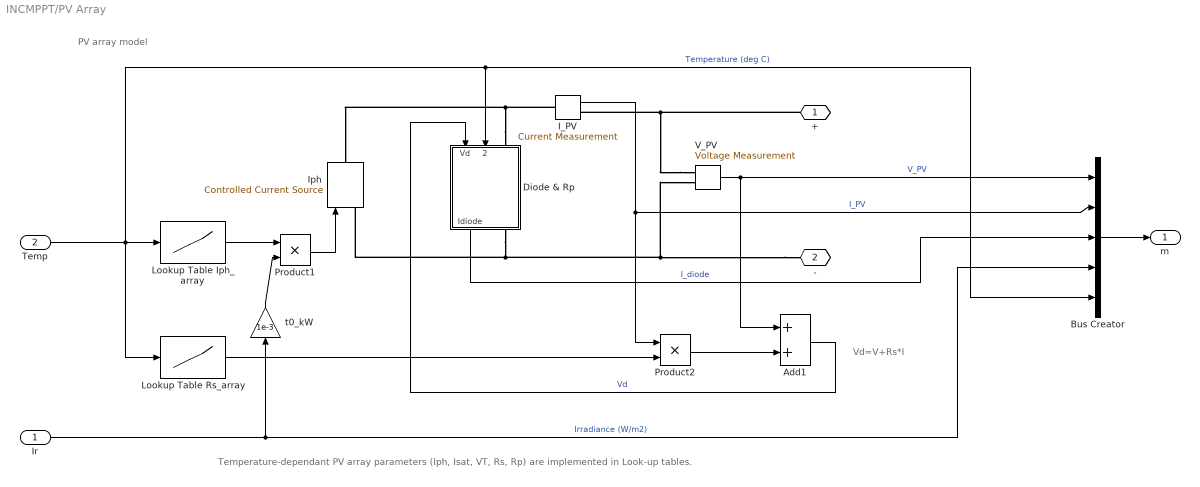
== system INCMPPT/PV Array ==
  note: Temperature-dependant PV array parameters (Iph, Isat, VT, Rs, Rp) are implemented in Look-up tables.
  note: Vd=V+Rs*I
  note: PV array model
  Ir : Inport
  Temp : Inport  Port=2
  Add1 : Sum
  Bus Creator : BusCreator  Inputs=5
  Diode & Rp : Subsystem
      mask Display:
      | plot(-75,-50,100,150, [-15 -15 43 -15 -15 -75],[50 8 50 92 50 50], ...
      |     [43 43],[8 94],[100 43], [50 50])
  I_PV : powerlib/Measurements/Current Measurement  PhasorSimulation=off  OutputType=Complex  PSBequivalent=0
  Iph : powerlib/Electrical Sources/Controlled Current Source  Initialize=on  Source_Type=AC  Amplitude=0  Phase=0  Frequency=0  Measurements=None
  Lookup Table Iph_array : Lookup_n-D  NumberOfTableDimensions=1  BreakpointsForDimension1=TempC  Table=Iph_array  RndMeth=Simplest  InputSameDT=on
  Lookup Table Rs_array : Lookup_n-D  NumberOfTableDimensions=1  BreakpointsForDimension1=TempC  Table=Rs_array  RndMeth=Simplest  InputSameDT=on
  Product1 : Product  Inputs=**  RndMeth=Zero
  Product2 : Product  Inputs=**  RndMeth=Zero
  V_PV : powerlib/Measurements/Voltage Measurement  PhasorSimulation=off  OutputType=Complex  PSBequivalent=0
  t0_kW : Gain  Gain=1e-3
  + : PMIOPort  Port=1  Side=Right
  - : PMIOPort  Port=2  Side=Right
  m : Outport
  wires:
  Add1/1 -> Diode & Rp/1(Vd)  "Vd"
  Product2/1 -> Add1/2
  V_PV/1 -> Add1/1, Bus Creator/1  "V_PV"
  Diode & Rp/1(Idiode) -> Bus Creator/3  "I_diode"
  t0_kW/1 -> Product1/2
  I_PV/1 -> Product2/1, Bus Creator/2  "I_PV"
  Ir/1 -> t0_kW/1, Bus Creator/4  "Irradiance (W/m2)"
  Product1/1 -> Iph/1
  Temp/1 -> Lookup Table Rs_array/1, Bus Creator/5, Diode & Rp/2(TempC), Lookup Table Iph_array/1  "Temperature (deg C)"
  Lookup Table Iph_array/1 -> Product1/1
  Lookup Table Rs_array/1 -> Product2/2
  Bus Creator/1 -> m/1
  connections:
  V_PV/LConn1 -- I_PV/RConn1 -- +/RConn1
  Diode & Rp/LConn1 -- I_PV/LConn1 -- Iph/RConn1
  -/RConn1 -- Iph/LConn1 -- Diode & Rp/RConn1 -- V_PV/LConn2

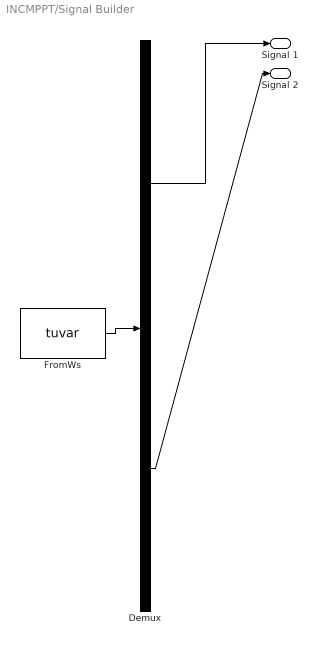
== system INCMPPT/Signal Builder ==
  Demux : Demux  Tag=STV Demux  Outputs=2
  FromWs : FromWorkspace  Tag=STV FromWs  VariableName=tuvar  SampleTime=0
      SigBuilderData=|
      | common.afterFinalStr = 'Extrapolate'
      | common.sampleTime = 0
      | dataSet.timeRange = [0 10]
      | dataSet.name = 'Group 1'
      | sbobj.Groups.Name = 'Group 1'
      | sbobj.Groups.Signals(1).Name = 'Signal 1'
      | sbobj.Groups.Signals(1).XData = [0 4 4 6 6 10]
      | sbobj.Groups.Signals(1).YData = [1000 1000 1 1 0 0]
      | sbobj.Groups.Signals(2).Name = 'Signal 2'
      | sbobj.Groups.Signals(2).XData = [0 10]
      | sbobj.Groups.Signals(2).YData = [25 25]
  Signal 1 : Outport  Tag=STV Outport
  Signal 2 : Outport  Tag=STV Outport  Port=2
  wires:
  Demux/1 -> Signal 1/1
  FromWs/1 -> Demux/1
  Demux/2 -> Signal 2/1

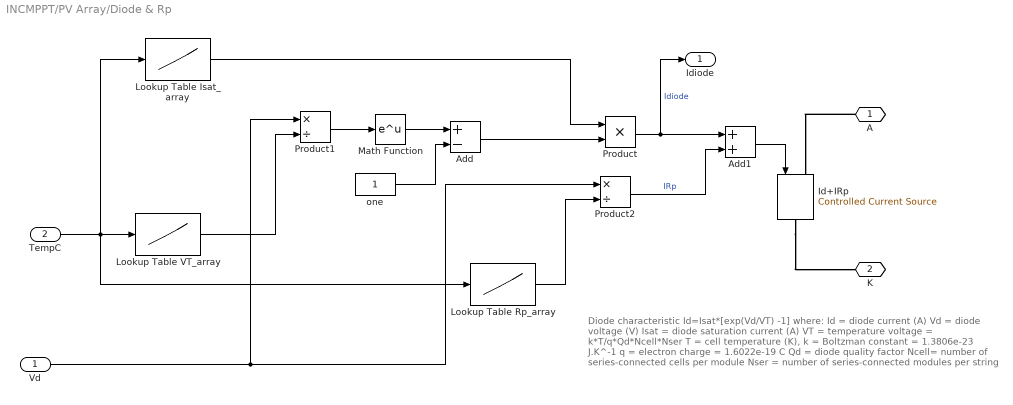
== system INCMPPT/PV Array/Diode & Rp ==
  note: Diode characteristic
      |    Id=Isat*[exp(Vd/VT) -1]
      |
      | where:
      |    Id = diode current (A)
      |    Vd = diode voltage (V)
      |  Isat = diode saturation current (A)
      |    VT = temperature voltage = k*T/q*Qd*Ncell*Nser
      |     T = cell temperature (K),
      |     k = Boltzman constant = 1.3806e-23 J.K^-1
      |     q = electron charge = 1.6022e-19 C
      |    Qd = diode quality factor
      |  Ncell= number of series-connected cells per module
      |  Nser = number of series-connected modules per string
  Vd : Inport
  TempC : Inport  Port=2
  Add : Sum  Inputs=+-
  Add1 : Sum
  Id+IRp : powerlib/Electrical Sources/Controlled Current Source  Initialize=on  Source_Type=AC  Amplitude=0  Phase=0  Frequency=0  Measurements=None
  Lookup Table Isat_array : Lookup_n-D  NumberOfTableDimensions=1  BreakpointsForDimension1=TempC  Table=Isat_array  RndMeth=Simplest  InputSameDT=on
  Lookup Table Rp_array : Lookup_n-D  NumberOfTableDimensions=1  BreakpointsForDimension1=TempC  Table=Rp_array  RndMeth=Simplest  InputSameDT=on
  Lookup Table VT_array : Lookup_n-D  NumberOfTableDimensions=1  BreakpointsForDimension1=TempC  Table=VT_array  RndMeth=Simplest  InputSameDT=on
  Math Function : Math  SaturateOnIntegerOverflow=on
  Product : Product  RndMeth=Zero
  Product1 : Product  Inputs=*/  RndMeth=Zero
  Product2 : Product  Inputs=*/  RndMeth=Zero
  one : Constant
  A : PMIOPort  Port=1  Side=Left
  K : PMIOPort  Port=2  Side=Right
  Idiode : Outport
  wires:
  Math Function/1 -> Add/1
  Vd/1 -> Product1/1, Product2/1
  Add1/1 -> Id+IRp/1
  Product2/1 -> Add1/2  "IRp"
  Product/1 -> Add1/1, Idiode/1  "Idiode"
  Product1/1 -> Math Function/1
  one/1 -> Add/2
  Add/1 -> Product/2
  Lookup Table VT_array/1 -> Product1/2
  TempC/1 -> Lookup Table Isat_array/1, Lookup Table VT_array/1, Lookup Table Rp_array/1
  Lookup Table Isat_array/1 -> Product/1
  Lookup Table Rp_array/1 -> Product2/2
  connections:
  Id+IRp/RConn1 -- K/RConn1
  A/RConn1 -- Id+IRp/LConn1

== matlab function INCMPPT/INC/MATLAB Function ==
  data: u input; y output; i input; uo input; io input; D input
function y = MYMPP(u,i,uo,io,D)
m=0.4;
du=u-uo;
di=i-io;
d=0.00005;
if du==0
    if di==0
    m=D;
    else
        if di>0
            m=D-d;
        else
            m=D+d;
        end
    end
else
    if di/du== -(i/u)
    m=D;
    else
        if di/du> -(i/u)
        m=D-d;
        else
            m=D+d;
        end
    end
end
y = m;
end
